simulink model "chap11_1sim"  (R2020a)
settings: Solver=VariableStepAuto  StartTime=0.0  StopTime=3  RelTol=1e-3
values from neighbouring files (symbols this model uses):
  C = [(-2*epc*sin(q2)+2*eta*cos(q2))*dq2   (-epc*sin(q2)+eta*cos(q2))*dq2 ... (first row only)    [chap11_1plant.m]
  m1 = 1    [chap11_1ctrl.m]    (also in chap11_1plant.m)
  q1 = u(7)    [chap11_1ctrl.m]    (also in chap11_1plant.m = x(1))
  q2 = u(9)    [chap11_1ctrl.m]    (also in chap11_1plant.m = x(3))
undefined symbols (not defined in the file or in its folder): c1, c2, c3, c4, del, delta3, delta4, DiscIntNeverNeededParam, g1, g2, g3, g4, gam, m2, m3, m4, mModel, q3, q4, Ts, z0
undefined symbols (not defined in the file): k
libraries: simulink x2
settings Model: Creator=khoi  LastModifiedBy=khoi

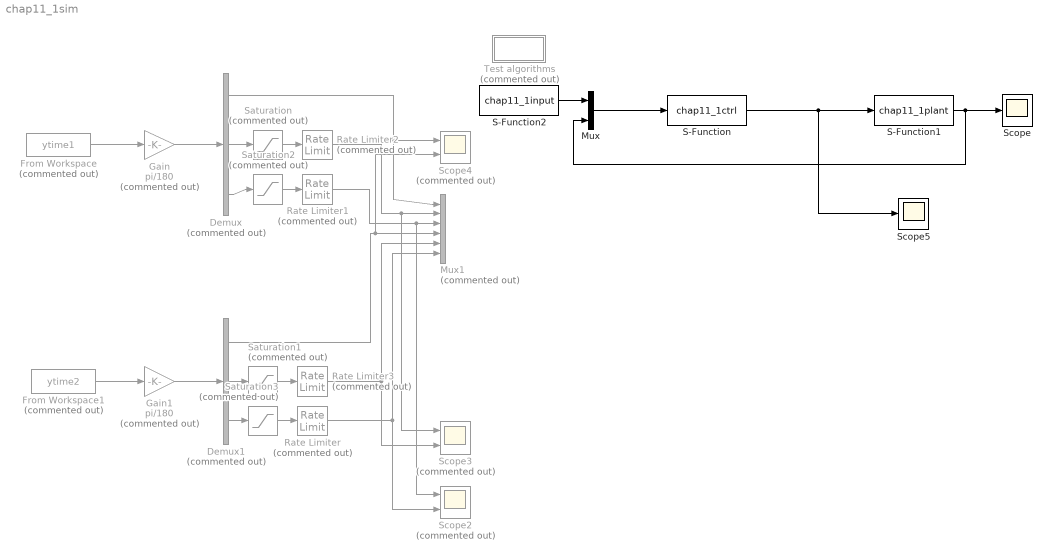
== system chap11_1sim ==
  Demux : Demux  Commented=on  Outputs=3
  Demux1 : Demux  Commented=on  Outputs=3
  From Workspace : FromWorkspace  Commented=on  VariableName=ytime1  SampleTime=Ts  OutputAfterFinalValue=Setting to zero
  From Workspace1 : FromWorkspace  Commented=on  VariableName=ytime2  SampleTime=Ts  OutputAfterFinalValue=Setting to zero
  Gain : Gain  Commented=on  Gain=pi/180
  Gain1 : Gain  Commented=on  Gain=pi/180
  Mux : Mux  Inputs=2
  Mux1 : Mux  Commented=on  Inputs=6
  Rate Limiter : RateLimiter  Commented=on  RisingSlewLimit=1.5e4  FallingSlewLimit=-1.5e4  SampleTimeMode=inherited
  Rate Limiter1 : RateLimiter  Commented=on  RisingSlewLimit=1e4  FallingSlewLimit=-1e4  SampleTimeMode=inherited
  Rate Limiter2 : RateLimiter  Commented=on  RisingSlewLimit=1e3  FallingSlewLimit=-1e3  SampleTimeMode=inherited
  Rate Limiter3 : RateLimiter  Commented=on  RisingSlewLimit=2e3  FallingSlewLimit=-2e3  SampleTimeMode=inherited
  S-Function : S-Function  FunctionName=chap11_1ctrl  SFunctionDeploymentMode=off  EnableBusSupport=off
  S-Function1 : S-Function  FunctionName=chap11_1plant  SFunctionDeploymentMode=off  EnableBusSupport=off
  S-Function2 : S-Function  FunctionName=chap11_1input  SFunctionDeploymentMode=off  EnableBusSupport=off
  Saturation : Saturate  Commented=on  UpperLimit=500  LowerLimit=-500
  Saturation1 : Saturate  Commented=on  UpperLimit=500  LowerLimit=-500
  Saturation2 : Saturate  Commented=on  UpperLimit=5000  LowerLimit=-5000
  Saturation3 : Saturate  Commented=on  UpperLimit=5000  LowerLimit=-5000
  Scope : Scope
  Scope2 : Scope  Commented=on  NumInputPorts=2
  Scope3 : Scope  Commented=on  NumInputPorts=2
  Scope4 : Scope  Commented=on  NumInputPorts=2
  Scope5 : Scope
  Test algorithms : Subsystem  Commented=on
  wires:
  From Workspace/1 -> Gain/1
  From Workspace1/1 -> Gain1/1
  Demux1/3 -> Saturation3/1
  Demux/3 -> Saturation2/1
  Demux/2 -> Saturation/1
  Demux1/2 -> Saturation1/1
  Demux/1 -> Scope4/1, Mux1/1
  Rate Limiter2/1 -> Scope3/1, Mux1/2
  Rate Limiter1/1 -> Scope2/1, Mux1/3
  Demux1/1 -> Scope4/2, Mux1/4
  Rate Limiter3/1 -> Mux1/5, Scope3/2
  Rate Limiter/1 -> Mux1/6, Scope2/2
  Saturation/1 -> Rate Limiter2/1
  Saturation1/1 -> Rate Limiter3/1
  Saturation2/1 -> Rate Limiter1/1
  Saturation3/1 -> Rate Limiter/1
  Mux/1 -> S-Function/1
  Gain/1 -> Demux/1
  Gain1/1 -> Demux1/1
  S-Function/1 -> Scope5/1, S-Function1/1
  S-Function1/1 -> Mux/2, Scope/1
  S-Function2/1 -> Mux/1

== system chap11_1sim/Test algorithms ==
  Controller : Subsystem
      settings: PortSchema="{\"entries\":[{\"content\":{\"sides\":[{\"content\":{\"connectorIds\":[\"In1\",\"In2\"]},\"type\":\"ConnectorPlacement.EquallySpacedRectSide\",\"uuid\":\"ab92a86c-b21c-4625-bceb-c2ca4b22964e\"},{\"content\":{\"connectorIds\":[\"Out1\"],\"side\":\"RIGHT\"},\"type\":\"ConnectorPlacement.EquallySpacedRectSide\",\"uuid\":\"86d5470f-e70b-4cc8-bc91-304fe436d503\"},{\"content\":{\"connectorIds\":[\"In3\"],\"side\":\"TOP\"},\"type\":\"ConnectorPlacement.EquallySpacedRectSide\",\"uuid\":\"909d1e71-533f-4362-b6db-886603c1c7d0\"}]},\"type\":\"ConnectorPlacement.EquallySpacedConnector\",\"uuid\":\"70811cc5-df37-4d12-bd38-ee8baa36081e\"}],\"packageUris\":[\"http://schema.mathworks.com/mf0/Connector/19700101\"],\"version\":\"1.0\"}"
  Subsystem : Subsystem
  Subsystem1 : Subsystem
  Subsystem2 : Subsystem
  Subsystem3 : Subsystem
  Subsystem4 : Subsystem

== system chap11_1sim/Test algorithms/Controller ==
  In Bus Element4 : Inport  PortName=desIn  Element=m
  In Bus Element : Inport  Port=2  PortName=stateIn  Element=X
  d(k) : Inport  Port=3
  Subsystem1 : Subsystem  Commented=on  mask{A=mModel{2,3}.A, B=mModel{2,3}.B, C=C(:,2), g=g2, q=q2, eta=m2, phi=c2, Ts=Ts}
      mask prompts: A "state space A"; B "state space B"; C "state space C"; g "SMC param 1 - g"; q "SMC param 2 - q"; eta "SMC param 3 - eta"; phi "Bounded thickness - phi"; Ts "Sample time"
      mask DialogControl Container3 Prompt: SMC param
  Subsystem2 : Subsystem  Commented=on  mask{A=mModel{3,3}.A, B=mModel{3,3}.B, C=C(:,3), g=g3, q=q3, m=m3, delta=delta3, phi=c3, Ts=Ts}
      mask prompts: A "state space A"; B "state space B"; C "state space C"; g "SMC param 1 - g"; q "SMC param 2 - q"; m "SMC param 3 - m"; delta "SMC param 4 - delta"; phi "Bounded thickness - phi"; Ts "Sample time"
      mask DialogControl Container3 Prompt: SMC param
  Subsystem3 : Subsystem  Commented=on  mask{A=mModel{4,3}.A, B=mModel{4,3}.B, C=C(:,4), g=g4, q=q4, eta=m4, phi=c4, Ts=Ts}
      mask prompts: A "state space A"; B "state space B"; C "state space C"; g "SMC param 1 - g"; q "SMC param 2 - q"; eta "SMC param 3 - eta"; phi "Bounded thickness - phi"; Ts "Sample time"
      mask DialogControl Container3 Prompt: SMC param
  Subsystem3s : Subsystem  Commented=on  mask{A=mModel{4,3}.A, B=mModel{4,3}.B, C=C(:,4), g=g4, q=q4, m=m4, delta=delta4, phi=c4, Ts=Ts}
      mask prompts: A "state space A"; B "state space B"; C "state space C"; g "SMC param 1 - g"; q "SMC param 2 - q"; m "SMC param 3 - m"; delta "SMC param 4 - delta"; phi "Bounded thickness - phi"; Ts "Sample time"
      mask DialogControl Container3 Prompt: SMC param
  Subsystem4 : Subsystem  Commented=on  mask{A=mModel{1,3}.A, B=mModel{1,3}.B, C=C(:,1), g=g1, q=q1, eta=m1, phi=c1, Ts=Ts}
      mask prompts: A "state space A"; B "state space B"; C "state space C"; g "SMC param 1 - g"; q "SMC param 2 - q"; eta "SMC param 3 - eta"; phi "Bounded thickness - phi"; Ts "Sample time"
      mask DialogControl Container3 Prompt: SMC param
  Out Bus Element : Outport  PortName=u(k)  Element=u(k)

== system chap11_1sim/Test algorithms/Subsystem ==
  Subsystem1 : Subsystem  mask{A=0, B=0, C=0, q=0, T=0, lam=0, gamm=0, vphi=0, bet=0}
      mask prompts: A "A discrete"; B "B discrete"; C "C sliding param"; q "convergence gain >0"; T "sample time"; lam "lambda > 0"; gamm "gamma > 0"; vphi "varphi > 0"; bet "0< beta <1"
      mask DialogControl ParameterGroupVar Prompt: State
      mask DialogControl ParameterGroupVar_copy Prompt: Exponential term

== system chap11_1sim/Test algorithms/Subsystem1 ==
  note: discrete-time variable structure controller with a decoupled disturbance compensator and its application to a CNC servomechanism
  Discrete State-Space : DiscreteStateSpace  A=[1 0.0006; 0 0.3074]  B=[0.0004; 0.6926]  C=eye(2)  D=[0;0]  SampleTime=-1
  Discrete-Time Integrator1 : DiscreteIntegrator  SampleTime=-1  ICPrevOutput=DiscIntNeverNeededParam  ICPrevScaledInput=DiscIntNeverNeededParam
  Gain2 : Gain  Gain=pi/30
  Mux : Mux  Inputs=2
  Step : Step  After=1200  SampleTime=0.001
  Subsystem : Subsystem  mask{A=[1 0.0006; 0 0.3074], B=[0.0004; 0.6926], C=[210; 1], eta=1.5854, phi=2.5, q=1, g=0.0159}
  wires:
  Discrete State-Space/1 -> Subsystem/2(In2)
  Mux/1 -> Subsystem/1(In1)
  Step/1 -> Mux/2, Gain2/1
  Gain2/1 -> Discrete-Time Integrator1/1
  Discrete-Time Integrator1/1 -> Mux/1
  Subsystem/1(Out1) -> Discrete State-Space/1

== system chap11_1sim/Test algorithms/Subsystem2 ==
  note: Test for-loop delay vector. Temporarily it is replaced by tapped delay block
  Add1 : Sum  Inputs=+++
  Constant : Constant
  Constant1 : Constant  Value=2
  Delay : Delay  DelayLengthSource=Input port  InitialCondition=0
      settings: InputPortMap=u0,p1
  Delay1 : Delay  DelayLengthSource=Input port  InitialCondition=0
      settings: InputPortMap=u0,p1
  Repeating Sequence Stair : simulink/Sources/Repeating Sequence Stair  OutValues=[0 1 2 3 4 5].'/10  tsamp=0.01  OutMin=[]  OutMax=[]  OutDataTypeStr=double  OutputDataTypeScalingMode=double  OutDataType=fixdt(0,8)  ConRadixGroup=Best Precision: Vector-wise  OutScaling=2^-12
  Scope4 : Scope  NumInputPorts=2
  wires:
  Constant/1 -> Delay/2
  Repeating Sequence Stair/1 -> Delay1/1, Delay/1, Add1/1
  Add1/1 -> Scope4/2
  Constant1/1 -> Delay1/2
  Delay/1 -> Add1/2
  Delay1/1 -> Add1/3

== system chap11_1sim/Test algorithms/Subsystem3 ==
  Discrete-Time Integrator : DiscreteIntegrator  Commented=on  IntegratorMethod=Integration: Backward Euler  SampleTime=-1  ICPrevOutput=DiscIntNeverNeededParam  ICPrevScaledInput=DiscIntNeverNeededParam
  Gain : Gain  Commented=on  Gain=gam
  Gain1 : Gain  Commented=on  Gain=eps
  MATLAB Function : MATLAB Function  Commented=on  TreatAsAtomicUnit=on
  MATLAB Function1 : MATLAB Function  Commented=on  TreatAsAtomicUnit=on  mask{c1=0, bet=0, gam=0, eps=0, the=0, rho=0, W=0, kP=0, Mbar=0, khat0=0, tauL=0, tautde0=0}
      mask prompts: bet "beta"; gam "gamma"; eps "epsilon"; the "theta"
  Sum : Sum  Commented=on  Inputs=|+-
  Unit Delay : UnitDelay  Commented=on  SampleTime=-1  HasFrameUpgradeWarning=on
  wires:
  Sum/1 -> Gain/1
  Discrete-Time Integrator/1 -> Unit Delay/1
  Unit Delay/1 -> Gain1/1
  Gain/1 -> Discrete-Time Integrator/1
  MATLAB Function1/1(sig) -> Sum/1
  Gain1/1 -> Sum/2

== system chap11_1sim/Test algorithms/Subsystem4 ==
  note: A novel dead zone reaching law of DSMC with disturbance compensation
  Scope5 : Scope
  Subsystem1 : Subsystem  mask{dsys=ss([1.2 0.1;0 0.6],[0;1],eye(2),[0;0]), C=[10 1], Ts=0.01, vphi=20, gamm=10, delt=0.38, qT=0.6, xiT=1e-10, eta=0.001, N=9}
      mask prompts: dsys "model"; vphi "varphi"; gamm "gamma"; delt "delta"
  Subsystem2 : Subsystem
  wires:
  Subsystem1/1(uk) -> Subsystem2/1(uk)
  Subsystem2/1(Out1) -> Subsystem1/1(In1), Scope5/1  "e(k)"

== system chap11_1sim/Test algorithms/Controller/Subsystem1 ==
  desIn : Inport
  stateIn : Inport  Port=2
  Add1 : Sum
  Rate Transition : RateTransition  OutPortSampleTime=Ts
  Rate Transition1 : RateTransition  OutPortSampleTime=Ts
  Saturation : Saturate  UpperLimit=2000  LowerLimit=-2000
  Subsystem : Subsystem
  Subsystem1 : Subsystem
  ctrlIn : Outport
  wires:
  Rate Transition/1 -> Subsystem1/1(Xd(k))
  Rate Transition1/1 -> Subsystem1/2(X(k))
  Subsystem1/1(us(k)) -> Add1/1  "us(k)"
  Subsystem1/2(s(k)) -> Subsystem/1(s(k))
  Add1/1 -> Saturation/1  "u(k)"
  Subsystem/1(uc(k)) -> Add1/2  "uc(k)"
  desIn/1 -> Rate Transition/1  "Xd(k)"
  stateIn/1 -> Rate Transition1/1  "X(k)"
  Saturation/1 -> ctrlIn/1

== system chap11_1sim/Test algorithms/Controller/Subsystem2 ==
  desIn : Inport
  stateIn : Inport  Port=2
  Add1 : Sum
  Rate Transition : RateTransition  OutPortSampleTime=Ts
  Rate Transition1 : RateTransition  OutPortSampleTime=Ts
  Subsystem : Subsystem
  Subsystem1 : Subsystem
  ctrlIn : Outport
  wires:
  stateIn/1 -> Rate Transition1/1  "X(k)"
  desIn/1 -> Rate Transition/1  "Xd(k)"
  Subsystem/1(uc(k)) -> Add1/2  "uc(k)"
  Add1/1 -> ctrlIn/1  "u(k)"
  Subsystem1/2(s(k)) -> Subsystem/1(s(k))
  Subsystem1/1(us(k)) -> Add1/1  "us(k)"
  Rate Transition1/1 -> Subsystem1/2(X(k))
  Rate Transition/1 -> Subsystem1/1(Xd(k))

== system chap11_1sim/Test algorithms/Controller/Subsystem3 ==
  desIn : Inport
  stateIn : Inport  Port=2
  Add1 : Sum
  Rate Transition : RateTransition  OutPortSampleTime=Ts
  Rate Transition1 : RateTransition  OutPortSampleTime=Ts
  Saturation : Saturate  UpperLimit=2000  LowerLimit=-2000
  Subsystem : Subsystem
  Subsystem1 : Subsystem
  ctrlIn : Outport
  wires:
  Saturation/1 -> ctrlIn/1
  stateIn/1 -> Rate Transition1/1  "X(k)"
  desIn/1 -> Rate Transition/1  "Xd(k)"
  Subsystem/1(uc(k)) -> Add1/2  "uc(k)"
  Add1/1 -> Saturation/1  "u(k)"
  Subsystem1/2(s(k)) -> Subsystem/1(s(k))
  Subsystem1/1(us(k)) -> Add1/1  "us(k)"
  Rate Transition1/1 -> Subsystem1/2(X(k))
  Rate Transition/1 -> Subsystem1/1(Xd(k))

== system chap11_1sim/Test algorithms/Controller/Subsystem3s ==
  desIn : Inport
  stateIn : Inport  Port=2
  Add1 : Sum
  Rate Transition : RateTransition  OutPortSampleTime=Ts
  Rate Transition1 : RateTransition  OutPortSampleTime=Ts
  Subsystem : Subsystem
  Subsystem1 : Subsystem
  ctrlIn : Outport
  wires:
  Rate Transition/1 -> Subsystem1/1(Xd(k))
  Rate Transition1/1 -> Subsystem1/2(X(k))
  Subsystem1/1(us(k)) -> Add1/1  "us(k)"
  Subsystem1/2(s(k)) -> Subsystem/1(s(k))
  Add1/1 -> ctrlIn/1  "u(k)"
  Subsystem/1(uc(k)) -> Add1/2  "uc(k)"
  desIn/1 -> Rate Transition/1  "Xd(k)"
  stateIn/1 -> Rate Transition1/1  "X(k)"

== system chap11_1sim/Test algorithms/Controller/Subsystem4 ==
  desIn : Inport
  stateIn : Inport  Port=2
  Add1 : Sum
  Rate Transition : RateTransition  OutPortSampleTime=Ts
  Rate Transition1 : RateTransition  OutPortSampleTime=Ts
  Saturation : Saturate  UpperLimit=2000  LowerLimit=-2000
  Subsystem : Subsystem
  Subsystem1 : Subsystem
  ctrlIn : Outport
  wires:
  Saturation/1 -> ctrlIn/1
  stateIn/1 -> Rate Transition1/1  "X(k)"
  desIn/1 -> Rate Transition/1  "Xd(k)"
  Subsystem/1(uc(k)) -> Add1/2  "uc(k)"
  Add1/1 -> Saturation/1  "u(k)"
  Subsystem1/2(s(k)) -> Subsystem/1(s(k))
  Subsystem1/1(us(k)) -> Add1/1  "us(k)"
  Rate Transition1/1 -> Subsystem1/2(X(k))
  Rate Transition/1 -> Subsystem1/1(Xd(k))

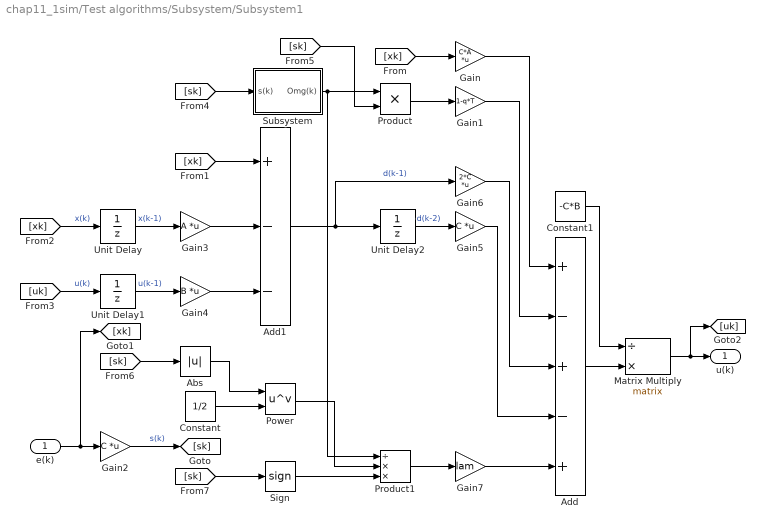
== system chap11_1sim/Test algorithms/Subsystem/Subsystem1 ==
  e(k) : Inport
  Abs : Abs
  Add : Sum  Inputs=+-+-+
  Add1 : Sum  Inputs=+--
  Constant : Constant  Value=1/2
  Constant1 : Constant  Value=-C*B
  Gain : Gain  Gain=C*A  Multiplication=Matrix(K*u) (u vector)
  Gain1 : Gain  Gain=1-q*T
  Gain2 : Gain  Gain=C  Multiplication=Matrix(K*u) (u vector)
  Gain3 : Gain  Gain=A  Multiplication=Matrix(K*u) (u vector)
  Gain4 : Gain  Gain=B  Multiplication=Matrix(K*u) (u vector)
  Gain5 : Gain  Gain=C  Multiplication=Matrix(K*u) (u vector)
  Gain6 : Gain  Gain=2*C  Multiplication=Matrix(K*u) (u vector)
  Gain7 : Gain  Gain=lam
  Matrix Multiply : Product  Inputs=/*  Multiplication=Matrix(*)
  Power : Math  Operator=pow  SaturateOnIntegerOverflow=on
  Product : Product
  Product1 : Product  Inputs=/**
  Sign : Signum
  Subsystem : Subsystem
  Unit Delay : UnitDelay  SampleTime=-1  HasFrameUpgradeWarning=on
  Unit Delay1 : UnitDelay  SampleTime=-1  HasFrameUpgradeWarning=on
  Unit Delay2 : UnitDelay  SampleTime=-1  HasFrameUpgradeWarning=on
  u(k) : Outport
  wires:
  Product1/1 -> Gain7/1
  Gain4/1 -> Add1/3
  Gain5/1 -> Add/4
  Abs/1 -> Power/1
  [sk] -> Subsystem/1(s(k))
  Add1/1 -> Unit Delay2/1, Gain6/1  "d(k-1)"
  Gain3/1 -> Add1/2
  [xk] -> Gain/1
  Gain1/1 -> Add/2
  [sk] -> Abs/1
  [xk] -> Unit Delay/1  "x(k)"
  Product/1 -> Gain1/1
  Unit Delay/1 -> Gain3/1  "x(k-1)"
  Sign/1 -> Product1/3
  [sk] -> Sign/1
  Subsystem/1(Omg(k)) -> Product/1, Product1/1
  [uk] -> Unit Delay1/1  "u(k)"
  Constant/1 -> Power/2
  Gain7/1 -> Add/5
  Add/1 -> Matrix Multiply/2
  Unit Delay1/1 -> Gain4/1  "u(k-1)"
  Constant1/1 -> Matrix Multiply/1
  [xk] -> Add1/1
  [sk] -> Product/2
  Unit Delay2/1 -> Gain5/1  "d(k-2)"
  Power/1 -> Product1/2
  Gain6/1 -> Add/3
  Gain/1 -> Add/1
  Gain2/1 -> [sk]  "s(k)"
  Matrix Multiply/1 -> u(k)/1, [uk]
  e(k)/1 -> Gain2/1, [xk]

== system chap11_1sim/Test algorithms/Subsystem1/Subsystem ==
  In1 : Inport
  In2 : Inport  Port=2
  Add1 : Sum  Inputs=+-
  Discrete-Time Integrator : DiscreteIntegrator  SampleTime=-1  ICPrevOutput=DiscIntNeverNeededParam  ICPrevScaledInput=DiscIntNeverNeededParam
  MATLAB Function : MATLAB Function  TreatAsAtomicUnit=on  mask{A=A, b=B, c=C, eta=eta, phi=phi, q=q}
  MATLAB Function1 : MATLAB Function  TreatAsAtomicUnit=on  mask{g=g, eta=eta, phi=phi, q=q, b=B, c=C}
  Rate Transition : RateTransition
  Rate Transition1 : RateTransition
  Unit Delay : UnitDelay  SampleTime=-1  HasFrameUpgradeWarning=on
  Unit Delay1 : UnitDelay  SampleTime=-1  HasFrameUpgradeWarning=on
  Out1 : Outport
  wires:
  Rate Transition/1 -> MATLAB Function/2(xrk), Discrete-Time Integrator/1
  MATLAB Function1/1(dk) -> Add1/2, Unit Delay1/1
  Rate Transition1/1 -> MATLAB Function/3(xk)
  MATLAB Function/2(sk) -> MATLAB Function1/1(sk), Unit Delay/1
  MATLAB Function/1(usk) -> Add1/1
  Unit Delay1/1 -> MATLAB Function1/3(dk_1)
  Discrete-Time Integrator/1 -> MATLAB Function/1(xrk1)
  In2/1 -> Rate Transition1/1  "X(k)"
  Unit Delay/1 -> MATLAB Function1/2(sk_1)
  In1/1 -> Rate Transition/1  "Xd(k)"
  Add1/1 -> Out1/1  "u(k)"

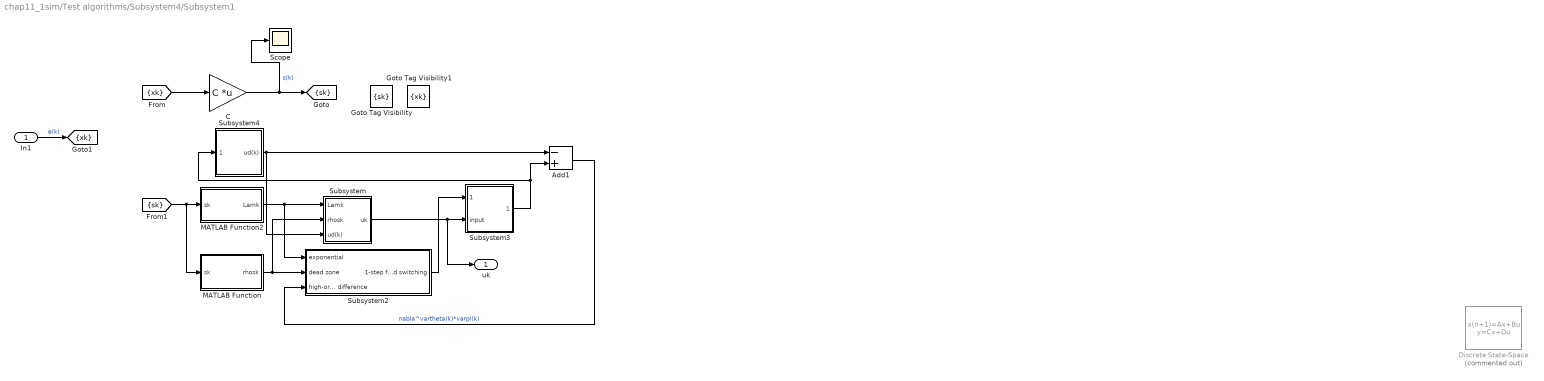
== system chap11_1sim/Test algorithms/Subsystem4/Subsystem1 ==
  In1 : Inport
  Add1 : Sum  Inputs=-+
  C : Gain  Gain=C  Multiplication=Matrix(K*u) (u vector)
  Discrete State-Space : DiscreteStateSpace  Commented=on  A=[1.2 0.1;0 0.6]  B=[0;1]  C=eye(2)  D=[0;0]  InitialCondition=[2;-6]  SampleTime=-1
  Goto Tag Visibility : GotoTagVisibility  GotoTag=sk
  Goto Tag Visibility1 : GotoTagVisibility  GotoTag=xk
  MATLAB Function : MATLAB Function  TreatAsAtomicUnit=on  mask{eta=eta}
      mask prompts: eta "eta>0"
  MATLAB Function2 : MATLAB Function  TreatAsAtomicUnit=on  mask{del=delt, vphi=vphi, gam=gamm}
      mask prompts: del "0<delta<1"; vphi "vphi>0"; gam "gamma>0 natrual number"
  Scope : Scope
  Subsystem : Subsystem
  Subsystem2 : Subsystem
  Subsystem3 : Subsystem
  Subsystem4 : Subsystem
  uk : Outport
  tag scope: sk=scoped, xk=scoped
  wires:
  In1/1 -> [xk]  "e(k)"
  C/1 -> Scope/1, [sk]  "s(k)"
  Subsystem4/1(ud(k)) -> Subsystem/3(ud(k)), Add1/1
  Subsystem2/1(1-step forward switching) -> Subsystem3/1(1-step forward switching)
  MATLAB Function/1(rhosk) -> Subsystem/2(rhosk), Subsystem2/2(dead zone)
  [xk] -> C/1
  Add1/1 -> Subsystem2/3(high-order difference)  "nabla^vartheta(k)*varpi(k)"
  Subsystem3/1(C*d(k)) -> Add1/2, Subsystem4/1(varpi(k))
  Subsystem/1(uk) -> uk/1, Subsystem3/2(input)
  MATLAB Function2/1(Lamk) -> Subsystem2/1(exponential), Subsystem/1(Lamk)
  [sk] -> MATLAB Function2/1(sk), MATLAB Function/1(sk)

== system chap11_1sim/Test algorithms/Subsystem4/Subsystem2 ==
  uk : Inport
  Constant : Constant  Value=0
  MATLAB Function : MATLAB Function  TreatAsAtomicUnit=on
  Mux : Mux  Inputs=2
  Sine Wave : Sin  Amplitude=2.5  Bias=0.157  Frequency=2*pi  SampleTime=0.01
  Unit Delay : UnitDelay  InitialCondition=[2;-6]  SampleTime=-1  HasFrameUpgradeWarning=on
  Out1 : Outport
  wires:
  Sine Wave/1 -> Mux/2
  Constant/1 -> Mux/1
  Mux/1 -> MATLAB Function/3(d)
  uk/1 -> MATLAB Function/1(u)
  MATLAB Function/1(dxk1) -> Unit Delay/1
  Unit Delay/1 -> Out1/1, MATLAB Function/2(xk)

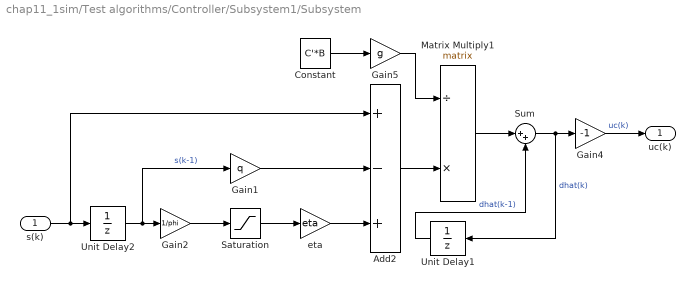
== system chap11_1sim/Test algorithms/Controller/Subsystem1/Subsystem ==
  s(k) : Inport
  Add2 : Sum  Inputs=+-+
  Constant : Constant  Value=C'*B
  Gain1 : Gain  Gain=q
  Gain2 : Gain  Gain=1/phi
  Gain4 : Gain  Gain=-1
  Gain5 : Gain  Gain=g
  Matrix Multiply1 : Product  Inputs=/*  Multiplication=Matrix(*)
  Saturation : Saturate  UpperLimit=1  LowerLimit=-1
  Sum : Sum  Inputs=|++
  Unit Delay1 : UnitDelay  SampleTime=-1  HasFrameUpgradeWarning=on
  Unit Delay2 : UnitDelay  SampleTime=-1  HasFrameUpgradeWarning=on
  eta : Gain  Gain=eta
  uc(k) : Outport
  wires:
  Constant/1 -> Gain5/1
  eta/1 -> Add2/3
  Add2/1 -> Matrix Multiply1/2
  Gain5/1 -> Matrix Multiply1/1
  Unit Delay1/1 -> Sum/2  "dhat(k-1)"
  Matrix Multiply1/1 -> Sum/1
  Gain1/1 -> Add2/2
  Gain2/1 -> Saturation/1
  Gain4/1 -> uc(k)/1  "uc(k)"
  Saturation/1 -> eta/1
  Unit Delay2/1 -> Gain1/1, Gain2/1  "s(k-1)"
  s(k)/1 -> Unit Delay2/1, Add2/1
  Sum/1 -> Gain4/1, Unit Delay1/1  "dhat(k)"

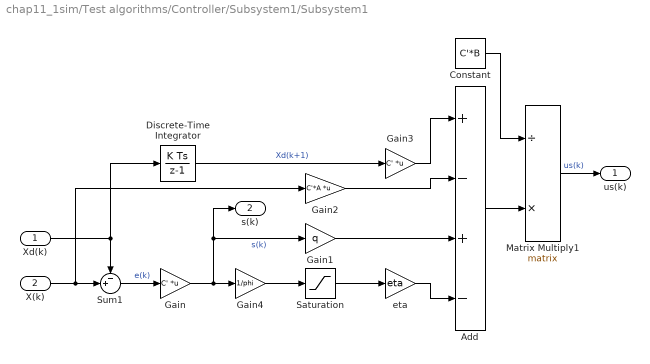
== system chap11_1sim/Test algorithms/Controller/Subsystem1/Subsystem1 ==
  Xd(k) : Inport
  X(k) : Inport  Port=2  PortDimensions=2
  Add : Sum  Inputs=+-+-
  Constant : Constant  Value=C'*B
  Discrete-Time Integrator : DiscreteIntegrator  SampleTime=-1  ICPrevOutput=DiscIntNeverNeededParam  ICPrevScaledInput=DiscIntNeverNeededParam
  Gain : Gain  Gain=C'  Multiplication=Matrix(K*u)
  Gain1 : Gain  Gain=q
  Gain2 : Gain  Gain=C'*A  Multiplication=Matrix(K*u)
  Gain3 : Gain  Gain=C'  Multiplication=Matrix(K*u)
  Gain4 : Gain  Gain=1/phi
  Matrix Multiply1 : Product  Inputs=/*  Multiplication=Matrix(*)
  Saturation : Saturate  UpperLimit=1  LowerLimit=-1
  Sum1 : Sum  Inputs=-+|
  eta : Gain  Gain=eta
  us(k) : Outport
  s(k) : Outport  Port=2
  wires:
  Add/1 -> Matrix Multiply1/2
  Gain2/1 -> Add/2
  Gain1/1 -> Add/3
  Constant/1 -> Matrix Multiply1/1
  X(k)/1 -> Sum1/2, Gain2/1
  Sum1/1 -> Gain/1  "e(k)"
  Discrete-Time Integrator/1 -> Gain3/1  "Xd(k+1)"
  Gain3/1 -> Add/1
  Saturation/1 -> eta/1
  Matrix Multiply1/1 -> us(k)/1  "us(k)"
  Gain4/1 -> Saturation/1
  eta/1 -> Add/4
  Xd(k)/1 -> Discrete-Time Integrator/1, Sum1/1
  Gain/1 -> Gain1/1, s(k)/1, Gain4/1  "s(k)"

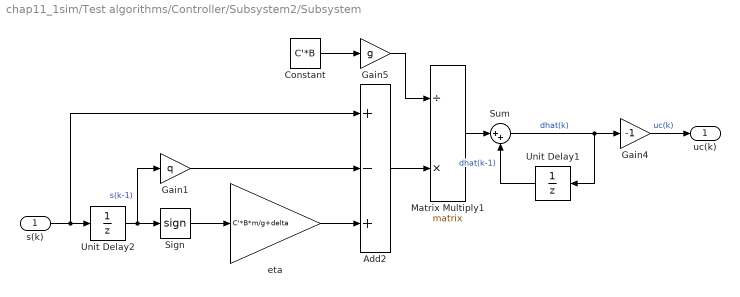
== system chap11_1sim/Test algorithms/Controller/Subsystem2/Subsystem ==
  s(k) : Inport
  Add2 : Sum  Inputs=+-+
  Constant : Constant  Value=C'*B
  Gain1 : Gain  Gain=q
  Gain4 : Gain  Gain=-1
  Gain5 : Gain  Gain=g
  Matrix Multiply1 : Product  Inputs=/*  Multiplication=Matrix(*)
  Sign : Signum
  Sum : Sum  Inputs=|++
  Unit Delay1 : UnitDelay  SampleTime=-1  HasFrameUpgradeWarning=on
  Unit Delay2 : UnitDelay  SampleTime=-1  HasFrameUpgradeWarning=on
  eta : Gain  Gain=C'*B*m/g+delta
  uc(k) : Outport
  wires:
  Add2/1 -> Matrix Multiply1/2
  Constant/1 -> Gain5/1
  Gain1/1 -> Add2/2
  Gain4/1 -> uc(k)/1  "uc(k)"
  Gain5/1 -> Matrix Multiply1/1
  Unit Delay1/1 -> Sum/2  "dhat(k-1)"
  Matrix Multiply1/1 -> Sum/1
  Sum/1 -> Unit Delay1/1, Gain4/1  "dhat(k)"
  Sign/1 -> eta/1
  eta/1 -> Add2/3
  s(k)/1 -> Add2/1, Unit Delay2/1
  Unit Delay2/1 -> Sign/1, Gain1/1  "s(k-1)"

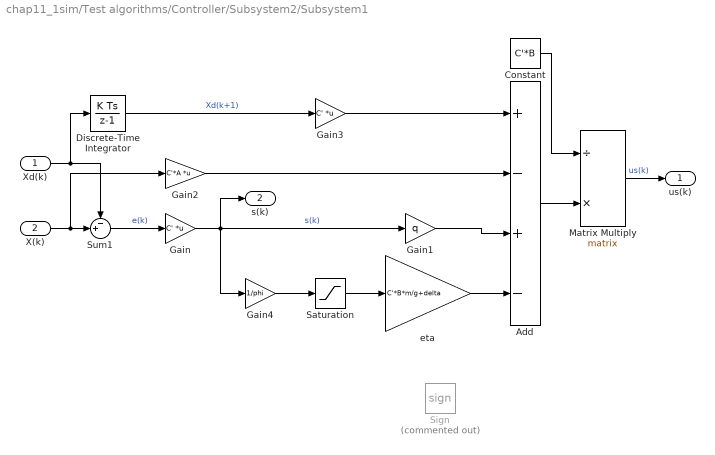
== system chap11_1sim/Test algorithms/Controller/Subsystem2/Subsystem1 ==
  Xd(k) : Inport
  X(k) : Inport  Port=2  PortDimensions=2
  Add : Sum  Inputs=+-+-
  Constant : Constant  Value=C'*B
  Discrete-Time Integrator : DiscreteIntegrator  SampleTime=-1  ICPrevOutput=DiscIntNeverNeededParam  ICPrevScaledInput=DiscIntNeverNeededParam
  Gain : Gain  Gain=C'  Multiplication=Matrix(K*u)
  Gain1 : Gain  Gain=q
  Gain2 : Gain  Gain=C'*A  Multiplication=Matrix(K*u)
  Gain3 : Gain  Gain=C'  Multiplication=Matrix(K*u)
  Gain4 : Gain  Gain=1/phi
  Matrix Multiply : Product  Inputs=/*  Multiplication=Matrix(*)
  Saturation : Saturate  UpperLimit=1  LowerLimit=-1
  Sign : Signum  Commented=on
  Sum1 : Sum  Inputs=-+|
  eta : Gain  Gain=C'*B*m/g+delta
  us(k) : Outport
  s(k) : Outport  Port=2
  wires:
  Gain4/1 -> Saturation/1
  eta/1 -> Add/4
  Gain2/1 -> Add/2
  Gain/1 -> s(k)/1, Gain4/1, Gain1/1  "s(k)"
  Constant/1 -> Matrix Multiply/1
  Gain3/1 -> Add/1
  Discrete-Time Integrator/1 -> Gain3/1  "Xd(k+1)"
  Add/1 -> Matrix Multiply/2
  Sum1/1 -> Gain/1  "e(k)"
  Gain1/1 -> Add/3
  Matrix Multiply/1 -> us(k)/1  "us(k)"
  Saturation/1 -> eta/1
  X(k)/1 -> Gain2/1, Sum1/2
  Xd(k)/1 -> Sum1/1, Discrete-Time Integrator/1

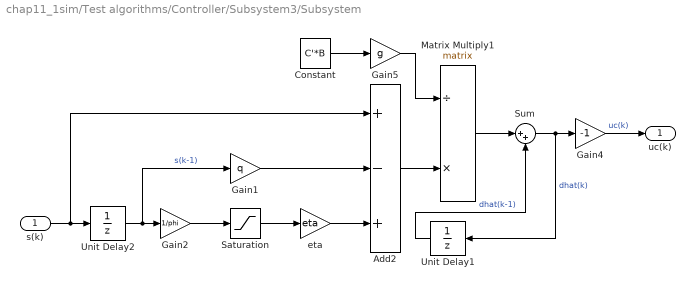
== system chap11_1sim/Test algorithms/Controller/Subsystem3/Subsystem ==
  s(k) : Inport
  Add2 : Sum  Inputs=+-+
  Constant : Constant  Value=C'*B
  Gain1 : Gain  Gain=q
  Gain2 : Gain  Gain=1/phi
  Gain4 : Gain  Gain=-1
  Gain5 : Gain  Gain=g
  Matrix Multiply1 : Product  Inputs=/*  Multiplication=Matrix(*)
  Saturation : Saturate  UpperLimit=1  LowerLimit=-1
  Sum : Sum  Inputs=|++
  Unit Delay1 : UnitDelay  SampleTime=-1  HasFrameUpgradeWarning=on
  Unit Delay2 : UnitDelay  SampleTime=-1  HasFrameUpgradeWarning=on
  eta : Gain  Gain=eta
  uc(k) : Outport
  wires:
  Sum/1 -> Unit Delay1/1, Gain4/1  "dhat(k)"
  s(k)/1 -> Add2/1, Unit Delay2/1
  Unit Delay2/1 -> Gain2/1, Gain1/1  "s(k-1)"
  Saturation/1 -> eta/1
  Gain4/1 -> uc(k)/1  "uc(k)"
  Gain2/1 -> Saturation/1
  Gain1/1 -> Add2/2
  Matrix Multiply1/1 -> Sum/1
  Unit Delay1/1 -> Sum/2  "dhat(k-1)"
  Gain5/1 -> Matrix Multiply1/1
  Add2/1 -> Matrix Multiply1/2
  eta/1 -> Add2/3
  Constant/1 -> Gain5/1

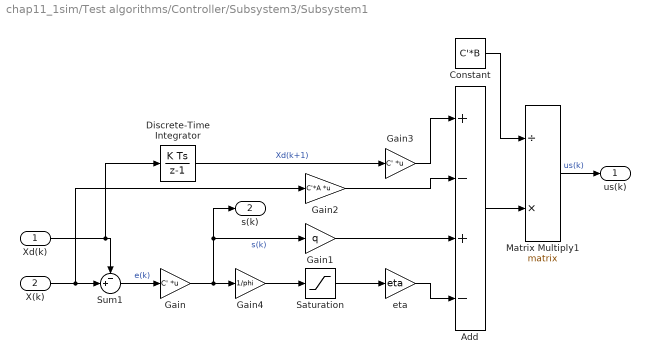
== system chap11_1sim/Test algorithms/Controller/Subsystem3/Subsystem1 ==
  Xd(k) : Inport
  X(k) : Inport  Port=2  PortDimensions=2
  Add : Sum  Inputs=+-+-
  Constant : Constant  Value=C'*B
  Discrete-Time Integrator : DiscreteIntegrator  SampleTime=-1  ICPrevOutput=DiscIntNeverNeededParam  ICPrevScaledInput=DiscIntNeverNeededParam
  Gain : Gain  Gain=C'  Multiplication=Matrix(K*u)
  Gain1 : Gain  Gain=q
  Gain2 : Gain  Gain=C'*A  Multiplication=Matrix(K*u)
  Gain3 : Gain  Gain=C'  Multiplication=Matrix(K*u)
  Gain4 : Gain  Gain=1/phi
  Matrix Multiply1 : Product  Inputs=/*  Multiplication=Matrix(*)
  Saturation : Saturate  UpperLimit=1  LowerLimit=-1
  Sum1 : Sum  Inputs=-+|
  eta : Gain  Gain=eta
  us(k) : Outport
  s(k) : Outport  Port=2
  wires:
  Gain/1 -> Gain4/1, s(k)/1, Gain1/1  "s(k)"
  Xd(k)/1 -> Sum1/1, Discrete-Time Integrator/1
  eta/1 -> Add/4
  Gain4/1 -> Saturation/1
  Matrix Multiply1/1 -> us(k)/1  "us(k)"
  Saturation/1 -> eta/1
  Gain3/1 -> Add/1
  Discrete-Time Integrator/1 -> Gain3/1  "Xd(k+1)"
  Sum1/1 -> Gain/1  "e(k)"
  X(k)/1 -> Gain2/1, Sum1/2
  Constant/1 -> Matrix Multiply1/1
  Gain1/1 -> Add/3
  Gain2/1 -> Add/2
  Add/1 -> Matrix Multiply1/2

== system chap11_1sim/Test algorithms/Controller/Subsystem3s/Subsystem ==
  s(k) : Inport
  Add2 : Sum  Inputs=+-+
  Constant : Constant  Value=C'*B
  Gain1 : Gain  Gain=q
  Gain4 : Gain  Gain=-1
  Gain5 : Gain  Gain=g
  Matrix Multiply1 : Product  Inputs=/*  Multiplication=Matrix(*)
  Sign : Signum
  Sum : Sum  Inputs=|++
  Unit Delay1 : UnitDelay  SampleTime=-1  HasFrameUpgradeWarning=on
  Unit Delay2 : UnitDelay  SampleTime=-1  HasFrameUpgradeWarning=on
  eta : Gain  Gain=C'*B*m/g+delta
  uc(k) : Outport
  wires:
  Unit Delay2/1 -> Gain1/1, Sign/1  "s(k-1)"
  s(k)/1 -> Unit Delay2/1, Add2/1
  eta/1 -> Add2/3
  Sign/1 -> eta/1
  Sum/1 -> Gain4/1, Unit Delay1/1  "dhat(k)"
  Matrix Multiply1/1 -> Sum/1
  Unit Delay1/1 -> Sum/2  "dhat(k-1)"
  Gain5/1 -> Matrix Multiply1/1
  Gain4/1 -> uc(k)/1  "uc(k)"
  Gain1/1 -> Add2/2
  Constant/1 -> Gain5/1
  Add2/1 -> Matrix Multiply1/2

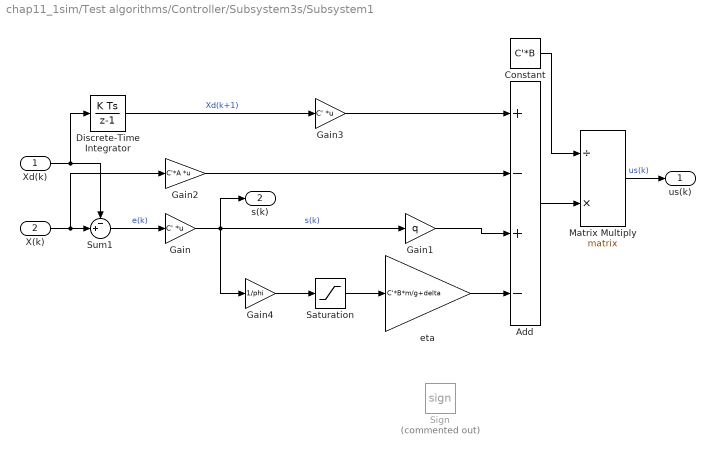
== system chap11_1sim/Test algorithms/Controller/Subsystem3s/Subsystem1 ==
  Xd(k) : Inport
  X(k) : Inport  Port=2  PortDimensions=2
  Add : Sum  Inputs=+-+-
  Constant : Constant  Value=C'*B
  Discrete-Time Integrator : DiscreteIntegrator  SampleTime=-1  ICPrevOutput=DiscIntNeverNeededParam  ICPrevScaledInput=DiscIntNeverNeededParam
  Gain : Gain  Gain=C'  Multiplication=Matrix(K*u)
  Gain1 : Gain  Gain=q
  Gain2 : Gain  Gain=C'*A  Multiplication=Matrix(K*u)
  Gain3 : Gain  Gain=C'  Multiplication=Matrix(K*u)
  Gain4 : Gain  Gain=1/phi
  Matrix Multiply : Product  Inputs=/*  Multiplication=Matrix(*)
  Saturation : Saturate  UpperLimit=1  LowerLimit=-1
  Sign : Signum  Commented=on
  Sum1 : Sum  Inputs=-+|
  eta : Gain  Gain=C'*B*m/g+delta
  us(k) : Outport
  s(k) : Outport  Port=2
  wires:
  Xd(k)/1 -> Discrete-Time Integrator/1, Sum1/1
  X(k)/1 -> Sum1/2, Gain2/1
  Saturation/1 -> eta/1
  Matrix Multiply/1 -> us(k)/1  "us(k)"
  Gain1/1 -> Add/3
  Sum1/1 -> Gain/1  "e(k)"
  Add/1 -> Matrix Multiply/2
  Discrete-Time Integrator/1 -> Gain3/1  "Xd(k+1)"
  Gain3/1 -> Add/1
  Constant/1 -> Matrix Multiply/1
  Gain/1 -> Gain1/1, Gain4/1, s(k)/1  "s(k)"
  Gain2/1 -> Add/2
  eta/1 -> Add/4
  Gain4/1 -> Saturation/1

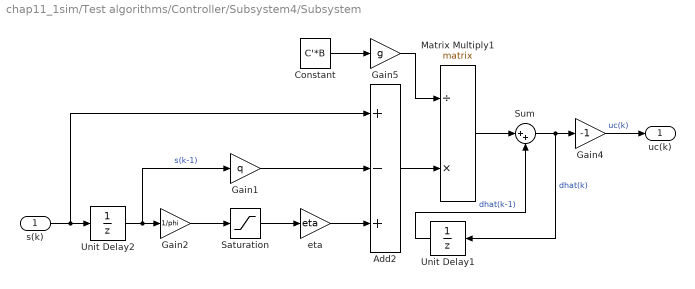
== system chap11_1sim/Test algorithms/Controller/Subsystem4/Subsystem ==
  s(k) : Inport
  Add2 : Sum  Inputs=+-+
  Constant : Constant  Value=C'*B
  Gain1 : Gain  Gain=q
  Gain2 : Gain  Gain=1/phi
  Gain4 : Gain  Gain=-1
  Gain5 : Gain  Gain=g
  Matrix Multiply1 : Product  Inputs=/*  Multiplication=Matrix(*)
  Saturation : Saturate  UpperLimit=1  LowerLimit=-1
  Sum : Sum  Inputs=|++
  Unit Delay1 : UnitDelay  SampleTime=-1  HasFrameUpgradeWarning=on
  Unit Delay2 : UnitDelay  SampleTime=-1  HasFrameUpgradeWarning=on
  eta : Gain  Gain=eta
  uc(k) : Outport
  wires:
  Sum/1 -> Unit Delay1/1, Gain4/1  "dhat(k)"
  s(k)/1 -> Add2/1, Unit Delay2/1
  Unit Delay2/1 -> Gain2/1, Gain1/1  "s(k-1)"
  Saturation/1 -> eta/1
  Gain4/1 -> uc(k)/1  "uc(k)"
  Gain2/1 -> Saturation/1
  Gain1/1 -> Add2/2
  Matrix Multiply1/1 -> Sum/1
  Unit Delay1/1 -> Sum/2  "dhat(k-1)"
  Gain5/1 -> Matrix Multiply1/1
  Add2/1 -> Matrix Multiply1/2
  eta/1 -> Add2/3
  Constant/1 -> Gain5/1

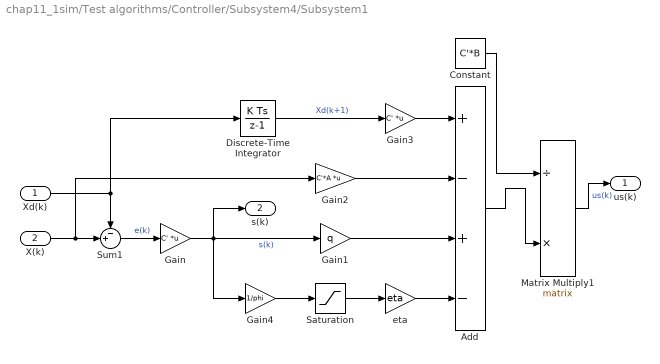
== system chap11_1sim/Test algorithms/Controller/Subsystem4/Subsystem1 ==
  Xd(k) : Inport
  X(k) : Inport  Port=2  PortDimensions=2
  Add : Sum  Inputs=+-+-
  Constant : Constant  Value=C'*B
  Discrete-Time Integrator : DiscreteIntegrator  SampleTime=-1  ICPrevOutput=DiscIntNeverNeededParam  ICPrevScaledInput=DiscIntNeverNeededParam
  Gain : Gain  Gain=C'  Multiplication=Matrix(K*u)
  Gain1 : Gain  Gain=q
  Gain2 : Gain  Gain=C'*A  Multiplication=Matrix(K*u)
  Gain3 : Gain  Gain=C'  Multiplication=Matrix(K*u)
  Gain4 : Gain  Gain=1/phi
  Matrix Multiply1 : Product  Inputs=/*  Multiplication=Matrix(*)
  Saturation : Saturate  UpperLimit=1  LowerLimit=-1
  Sum1 : Sum  Inputs=-+|
  eta : Gain  Gain=eta
  us(k) : Outport
  s(k) : Outport  Port=2
  wires:
  Xd(k)/1 -> Sum1/1, Discrete-Time Integrator/1
  X(k)/1 -> Gain2/1, Sum1/2
  Gain/1 -> s(k)/1, Gain4/1, Gain1/1  "s(k)"
  Saturation/1 -> eta/1
  Matrix Multiply1/1 -> us(k)/1  "us(k)"
  Gain1/1 -> Add/3
  Gain3/1 -> Add/1
  Discrete-Time Integrator/1 -> Gain3/1  "Xd(k+1)"
  Sum1/1 -> Gain/1  "e(k)"
  Constant/1 -> Matrix Multiply1/1
  Gain2/1 -> Add/2
  Add/1 -> Matrix Multiply1/2
  Gain4/1 -> Saturation/1
  eta/1 -> Add/4

== system chap11_1sim/Test algorithms/Subsystem/Subsystem1/Subsystem ==
  s(k) : Inport
  Abs : Abs
  Add : Sum
  Constant : Constant  Value=gamm
  Constant1 : Constant  Value=bet
  Exp : Math  SaturateOnIntegerOverflow=on
  Gain : Gain  Gain=-vphi
  Gain1 : Gain  Gain=(1-bet)
  Power : Math  Operator=pow  SaturateOnIntegerOverflow=on
  Omg(k) : Outport
  wires:
  Constant/1 -> Power/2
  Power/1 -> Gain/1
  s(k)/1 -> Abs/1
  Exp/1 -> Gain1/1
  Abs/1 -> Power/1
  Gain1/1 -> Add/2
  Constant1/1 -> Add/1
  Gain/1 -> Exp/1
  Add/1 -> Omg(k)/1

== system chap11_1sim/Test algorithms/Subsystem4/Subsystem1/Subsystem ==
  Lamk : Inport
  rhosk : Inport  Port=2
  ud(k) : Inport  Port=3
  Goto Tag Visibility : GotoTagVisibility  GotoTag=sk
  Goto Tag Visibility1 : GotoTagVisibility  GotoTag=xk
  MATLAB Function5 : MATLAB Function  TreatAsAtomicUnit=on  mask{Phi=dsys.A, Gam=dsys.B, C=C, qT=qT, xiT=xiT}
  uk : Outport
  wires:
  [sk] -> MATLAB Function5/2(sk)
  rhosk/1 -> MATLAB Function5/4(rhosk)
  Lamk/1 -> MATLAB Function5/3(Lamk)
  MATLAB Function5/1(uk) -> uk/1
  ud(k)/1 -> MATLAB Function5/5(udk)
  [xk] -> MATLAB Function5/1(xk)

== system chap11_1sim/Test algorithms/Subsystem4/Subsystem1/Subsystem2 ==
  exponential : Inport
  dead zone : Inport  Port=2
  high-order difference : Inport  Port=3
  Goto Tag Visibility : GotoTagVisibility  GotoTag=sk
  MATLAB Function1 : MATLAB Function  TreatAsAtomicUnit=on  mask{xiT=xiT, qT=qT}
      mask prompts: xiT "xi > 0 (xiT>0)"; qT "q (0<1-qT<1)"
  1-step forward switching : Outport
  wires:
  exponential/1 -> MATLAB Function1/2(Lamk)
  dead zone/1 -> MATLAB Function1/3(rhosk)
  high-order difference/1 -> MATLAB Function1/4(hodf)
  MATLAB Function1/1(sk1) -> 1-step forward switching/1  "s(k+1)"
  [sk] -> MATLAB Function1/1(sk)

== system chap11_1sim/Test algorithms/Subsystem4/Subsystem1/Subsystem3 ==
  1-step forward switching : Inport
  input : Inport  Port=2
  Add : Sum  Inputs=+--
  C*Gamma : Gain  Gain=C*dsys.B  Multiplication=Matrix(K*u)
  C*Phi : Gain  Gain=C*dsys.A  Multiplication=Matrix(K*u) (u vector)
  Goto Tag Visibility : GotoTagVisibility  GotoTag=xk
  C*d(k) : Outport
  wires:
  1-step forward switching/1 -> Add/1  "s(k+1)"
  [xk] -> C*Phi/1
  Add/1 -> C*d(k)/1  "C*d(k)"
  input/1 -> C*Gamma/1
  C*Phi/1 -> Add/2  "C*Phi*x(k)"
  C*Gamma/1 -> Add/3  "C*Gamma*u(k)"

== system chap11_1sim/Test algorithms/Subsystem4/Subsystem1/Subsystem4 ==
  varpi(k) : Inport
  Clock1 : Clock
  MATLAB Function3 : MATLAB Function  TreatAsAtomicUnit=on
  MATLAB Function4 : MATLAB Function  TreatAsAtomicUnit=on  mask{Ts=Ts, n=N}
  Rate Transition1 : RateTransition  OutPortSampleTime=Ts
  Tapped Delay : simulink/Discrete/Tapped Delay  vinit=0.0  samptime=-1  NumDelays=N  DelayOrder=Newest  includeCurrent=off
  ud(k) : Outport
  wires:
  MATLAB Function3/1(udk) -> ud(k)/1  "ud(k)"
  varpi(k)/1 -> Tapped Delay/1
  MATLAB Function4/1(vphik) -> MATLAB Function3/2(vthe)
  Rate Transition1/1 -> MATLAB Function4/1(t)
  Clock1/1 -> Rate Transition1/1
  Tapped Delay/1 -> MATLAB Function3/1(Cdk_i)

== matlab function chap11_1sim/Test algorithms/Subsystem4/Subsystem1/Subsystem/MATLAB Function5 ==
  data: xk input; uk output; sk input; Lamk input; rhosk input; udk input; Phi parameter; Gam parameter; C parameter; qT parameter; xiT parameter
function uk = fcn(xk,sk,Lamk,rhosk,udk,...
    Phi, Gam, C, qT, xiT)

uk = -(C*Gam)\(C*Phi*xk - (1-qT)*Lamk*sk + xiT/Lamk*rhosk + udk);

== matlab function chap11_1sim/Test algorithms/Subsystem4/Subsystem1/Subsystem2/MATLAB Function1 ==
  data: sk input; sk1 output; Lamk input; rhosk input; hodf input; xiT parameter; qT parameter
function sk1 = fFwrdSwit(sk,Lamk,rhosk,hodf,...
    xiT, qT)

sk1 = (1-qT)*Lamk*sk - xiT/Lamk*rhosk + hodf;

== matlab function chap11_1sim/Test algorithms/Subsystem4/Subsystem1/Subsystem4/MATLAB Function3 ==
  data: Cdk_i input; vthe input; udk output
function udk = fDtbCompen(Cdk_i,vthe)
udk = 0;
for i=1:vthe
    udk = udk - (-1)^i*nchoosek(vthe,i)*Cdk_i(i);
end

== matlab function chap11_1sim/Test algorithms/Subsystem4/Subsystem1/Subsystem4/MATLAB Function4 ==
  data: t input; vphik output; Ts parameter; n parameter
function vphik = fVphi(t,Ts,n)
persistent k;
if isempty(k)
    k=0;
end
if rem(t,Ts)==0 && t~=0 && k<n
    k = k+1;
end
vphik = k;

== matlab function chap11_1sim/Test algorithms/Subsystem4/Subsystem2/MATLAB Function ==
  data: u input; dxk1 output; xk input; d input
function dxk1 = fcn(u,xk,d)

dxk1 = [1.2 0.1;0 0.6]*xk + [0;1]*u + d;

== matlab function chap11_1sim/Test algorithms/Subsystem3/MATLAB Function1 ==
  data: dIn input; sIn input; c1 parameter; bet parameter; the parameter; sig output; z0 parameter; del parameter
function sig = fcn(dIn,sIn,...
    c1, bet, the, z0, del)
    z1 = sIn(1) - dIn(1);
    dz1 = sIn(2) - dIn(2);
    alp1 = -c1*z1 + dIn(2);
    z2 = sIn(2) - alp1;
    
    % sliding surface
    sigbar0 = z0(1) + bet*abs(z0(2))^del*sign(z0(2));
    sig = z1 + bet*z2^del*sign(z2)-exp(-the*t)*sigbar0;

== matlab function chap11_1sim/Test algorithms/Subsystem3/MATLAB Function ==
  data: u input; y output; gam input; eps input; rho input; W input; kP input; Mbar input; khat0 input; tauL input; tautde0 input
function y = fcn2(u,...
     gam, eps, rho, W, kP, Mbar, khat0, tauL, tautde0)
    
y = u;

== matlab function chap11_1sim/Test algorithms/Subsystem1/Subsystem/MATLAB Function ==
  data: xrk1 input; usk output; xrk input; xk input; A parameter; b parameter; c parameter; eta parameter; phi parameter; q parameter; sk output
function [usk,sk] = fusk(xrk1,xrk,xk,...
    A, b, c, eta, phi, q)
    sk = c'*(xk-xrk);
    saty = sk/phi;
    if abs(saty) > 1
        saty = sign(saty);
    end
    usk = (c'*b)\(c'*xrk1 - c'*A*xk + q*sk - eta*saty);

== matlab function chap11_1sim/Test algorithms/Subsystem1/Subsystem/MATLAB Function1 ==
  data: sk input; dk output; sk_1 input; dk_1 input; g parameter; eta parameter; phi parameter; q parameter; b parameter; c parameter
function dk = fudk(sk,sk_1,dk_1,...
    g, eta, phi, q, b, c)
    saty = sk_1/phi;
    if abs(saty)>1
        saty = sign(saty);
    end
    dk = dk_1 + g*(c'*b)\(sk - q*sk_1 + eta*saty);

== matlab function chap11_1sim/Test algorithms/Subsystem4/Subsystem1/MATLAB Function ==
  data: sk input; rhosk output; eta parameter
function rhosk = fDeadzone(sk,eta)
    if sk>eta
        rhosk=1;
    elseif abs(sk)<=eta
        rhosk=0;
    else % sk<-eta
        rhosk=-1;
    end

== matlab function chap11_1sim/Test algorithms/Subsystem4/Subsystem1/MATLAB Function2 ==
  data: sk input; Lamk output; del parameter; vphi parameter; gam parameter
function Lamk = fLambda(sk,del,vphi,gam)
Lamk= del + (1-del)*exp(-vphi*abs(sk)^gam);
